simulink model "LV25P_start"  (R2020b)
settings: Solver=VariableStepAuto  StartTime=0.0  StopTime=1/15  RelTol=1e-3
libraries: fl_lib x42, nesl_utility x17
settings Model: Creator=MrNobody  LastModifiedBy=david

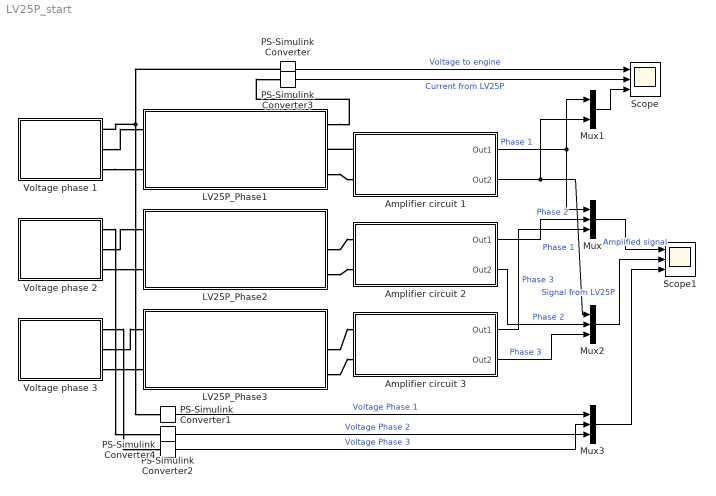
== system LV25P_start ==
  Amplifier circuit 1 : Subsystem
  Amplifier circuit 2 : Subsystem
  Amplifier circuit 3 : Subsystem
  LV25P_Phase1 : Subsystem
  LV25P_Phase2 : Subsystem
  LV25P_Phase3 : Subsystem
  Mux : Mux  Inputs=3
  Mux1 : Mux  Inputs=2
  Mux2 : Mux  Inputs=3
  Mux3 : Mux  Inputs=3
  PS-Simulink Converter{,1..4} (5 alike) : nesl_utility/PS-Simulink Converter  PhysicalDomain=network_engine_domain  SubClassName=ps_output  LeftPortType=input  RightPortType=output  PseudoPeriodic=off  Frequencies=[]  Unit=inherit  AffineConversion=off
  Scope : Scope  NumInputPorts=3
  Scope1 : Scope  NumInputPorts=3
  Voltage phase 1 : Subsystem
  Voltage phase 2 : Subsystem
  Voltage phase 3 : Subsystem
  wires:
  PS-Simulink Converter/1 -> Scope/1  "Voltage to engine"
  PS-Simulink Converter3/1 -> Scope/2  "Current from LV25P"
  Amplifier circuit 1/1(Out1) -> Mux1/1, Mux/1  "Phase 1"
  Amplifier circuit 2/1(Out1) -> Mux/2  "Phase 2"
  Amplifier circuit 3/1(Out1) -> Mux/3  "Phase 3"
  Mux/1 -> Scope1/1  "Amplified signal"
  Amplifier circuit 1/2(Out2) -> Mux2/1, Mux1/2  "Phase 1"
  Mux1/1 -> Scope/3
  Amplifier circuit 2/2(Out2) -> Mux2/2  "Phase 2"
  Amplifier circuit 3/2(Out2) -> Mux2/3  "Phase 3"
  Mux2/1 -> Scope1/2  "Signal from LV25P"
  PS-Simulink Converter4/1 -> Mux3/3  "Voltage Phase 3"
  PS-Simulink Converter2/1 -> Mux3/2  "Voltage Phase 2"
  PS-Simulink Converter1/1 -> Mux3/1  "Voltage Phase 1"
  Mux3/1 -> Scope1/3
  connections:
  PS-Simulink Converter/LConn1 -- Voltage phase 1/RConn1 -- PS-Simulink Converter1/LConn1
  Voltage phase 1/RConn2 -- LV25P_Phase1/LConn1
  Voltage phase 1/RConn3 -- LV25P_Phase1/LConn2
  LV25P_Phase1/RConn1 -- PS-Simulink Converter3/LConn1
  Amplifier circuit 1/LConn1 -- LV25P_Phase1/RConn2
  LV25P_Phase1/RConn3 -- Amplifier circuit 1/LConn2
  Voltage phase 2/RConn2 -- LV25P_Phase2/LConn1
  Voltage phase 2/RConn3 -- LV25P_Phase2/LConn2
  Voltage phase 3/RConn2 -- LV25P_Phase3/LConn1
  Voltage phase 3/RConn3 -- LV25P_Phase3/LConn2
  LV25P_Phase2/RConn2 -- Amplifier circuit 2/LConn1
  LV25P_Phase2/RConn3 -- Amplifier circuit 2/LConn2
  LV25P_Phase3/RConn2 -- Amplifier circuit 3/LConn1
  LV25P_Phase3/RConn3 -- Amplifier circuit 3/LConn2
  Voltage phase 3/RConn1 -- PS-Simulink Converter4/LConn1
  Voltage phase 2/RConn1 -- PS-Simulink Converter2/LConn1

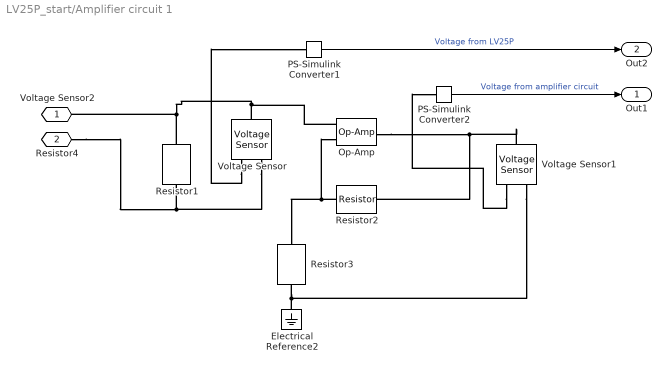
== system LV25P_start/Amplifier circuit 1 ==
  Electrical Reference2 : fl_lib/Electrical/Electrical Elements/Electrical Reference
  Op-Amp : fl_lib/Electrical/Electrical Elements/Op-Amp  outI_specify=off  outI_priority=None  outI=0 A  outI_nominal_specify=off  outI_nominal_unit=A  outI_nominal_value=1
  PS-Simulink Converter1 : nesl_utility/PS-Simulink Converter  PhysicalDomain=network_engine_domain  SubClassName=ps_output  LeftPortType=input  RightPortType=output  PseudoPeriodic=off  Frequencies=[]  Unit=inherit  AffineConversion=off
  PS-Simulink Converter2 : nesl_utility/PS-Simulink Converter  PhysicalDomain=network_engine_domain  SubClassName=ps_output  LeftPortType=input  RightPortType=output  PseudoPeriodic=off  Frequencies=[]  Unit=inherit  AffineConversion=off
  Resistor1 : fl_lib/Electrical/Electrical Elements/Resistor  R=100 Ohm  i_specify=off  i_priority=None  i=0 A  i_nominal_specify=off  i_nominal_unit=A  i_nominal_value=1  v_specify=off  v_priority=None  v=0 V  v_nominal_specify=off  v_nominal_unit=V  v_nominal_value=1
  Resistor2 : fl_lib/Electrical/Electrical Elements/Resistor  R=30 kOhm  i_specify=off  i_priority=None  i=0 A  i_nominal_specify=off  i_nominal_unit=A  i_nominal_value=1  v_specify=off  v_priority=None  v=0 V  v_nominal_specify=off  v_nominal_unit=V  v_nominal_value=1
  Resistor3 : fl_lib/Electrical/Electrical Elements/Resistor  R=10 kOhm  i_specify=off  i_priority=None  i=0 A  i_nominal_specify=off  i_nominal_unit=A  i_nominal_value=1  v_specify=off  v_priority=None  v=0 V  v_nominal_specify=off  v_nominal_unit=V  v_nominal_value=1
  Voltage Sensor : fl_lib/Electrical/Electrical Sensors/Voltage Sensor
  Voltage Sensor1 : fl_lib/Electrical/Electrical Sensors/Voltage Sensor
  Voltage Sensor2 : PMIOPort  Side=Left
  Resistor4 : PMIOPort  Port=2  Side=Left
  Out1 : Outport
  Out2 : Outport  Port=2
  wires:
  PS-Simulink Converter2/1 -> Out1/1  "Voltage from amplifier circuit"
  PS-Simulink Converter1/1 -> Out2/1  "Voltage from LV25P"
  connections:
  Resistor1/LConn1 -- Op-Amp/LConn1 -- Voltage Sensor/LConn1 -- Voltage Sensor2/RConn1
  Op-Amp/RConn1 -- Voltage Sensor1/LConn1 -- Resistor2/RConn1
  Voltage Sensor/RConn2 -- Resistor4/RConn1 -- Resistor1/RConn1
  Voltage Sensor1/RConn1 -- PS-Simulink Converter2/LConn1
  Electrical Reference2/LConn1 -- Voltage Sensor1/RConn2 -- Resistor3/RConn1
  Resistor2/LConn1 -- Op-Amp/LConn2 -- Resistor3/LConn1
  Voltage Sensor/RConn1 -- PS-Simulink Converter1/LConn1

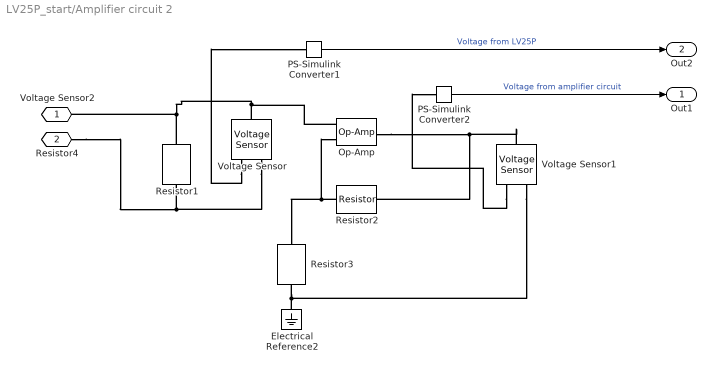
== system LV25P_start/Amplifier circuit 2 ==
  Electrical Reference2 : fl_lib/Electrical/Electrical Elements/Electrical Reference
  Op-Amp : fl_lib/Electrical/Electrical Elements/Op-Amp  outI_specify=off  outI_priority=None  outI=0 A  outI_nominal_specify=off  outI_nominal_unit=A  outI_nominal_value=1
  PS-Simulink Converter1 : nesl_utility/PS-Simulink Converter  PhysicalDomain=network_engine_domain  SubClassName=ps_output  LeftPortType=input  RightPortType=output  PseudoPeriodic=off  Frequencies=[]  Unit=inherit  AffineConversion=off
  PS-Simulink Converter2 : nesl_utility/PS-Simulink Converter  PhysicalDomain=network_engine_domain  SubClassName=ps_output  LeftPortType=input  RightPortType=output  PseudoPeriodic=off  Frequencies=[]  Unit=inherit  AffineConversion=off
  Resistor1 : fl_lib/Electrical/Electrical Elements/Resistor  R=100 Ohm  i_specify=off  i_priority=None  i=0 A  i_nominal_specify=off  i_nominal_unit=A  i_nominal_value=1  v_specify=off  v_priority=None  v=0 V  v_nominal_specify=off  v_nominal_unit=V  v_nominal_value=1
  Resistor2 : fl_lib/Electrical/Electrical Elements/Resistor  R=30 kOhm  i_specify=off  i_priority=None  i=0 A  i_nominal_specify=off  i_nominal_unit=A  i_nominal_value=1  v_specify=off  v_priority=None  v=0 V  v_nominal_specify=off  v_nominal_unit=V  v_nominal_value=1
  Resistor3 : fl_lib/Electrical/Electrical Elements/Resistor  R=10 kOhm  i_specify=off  i_priority=None  i=0 A  i_nominal_specify=off  i_nominal_unit=A  i_nominal_value=1  v_specify=off  v_priority=None  v=0 V  v_nominal_specify=off  v_nominal_unit=V  v_nominal_value=1
  Voltage Sensor : fl_lib/Electrical/Electrical Sensors/Voltage Sensor
  Voltage Sensor1 : fl_lib/Electrical/Electrical Sensors/Voltage Sensor
  Voltage Sensor2 : PMIOPort  Side=Left
  Resistor4 : PMIOPort  Port=2  Side=Left
  Out1 : Outport
  Out2 : Outport  Port=2
  wires:
  PS-Simulink Converter2/1 -> Out1/1  "Voltage from amplifier circuit"
  PS-Simulink Converter1/1 -> Out2/1  "Voltage from LV25P"
  connections:
  Op-Amp/LConn1 -- Voltage Sensor/LConn1 -- Resistor1/LConn1 -- Voltage Sensor2/RConn1
  Op-Amp/RConn1 -- Voltage Sensor1/LConn1 -- Resistor2/RConn1
  Voltage Sensor/RConn2 -- Resistor1/RConn1 -- Resistor4/RConn1
  Voltage Sensor1/RConn1 -- PS-Simulink Converter2/LConn1
  Electrical Reference2/LConn1 -- Voltage Sensor1/RConn2 -- Resistor3/RConn1
  Resistor2/LConn1 -- Op-Amp/LConn2 -- Resistor3/LConn1
  Voltage Sensor/RConn1 -- PS-Simulink Converter1/LConn1

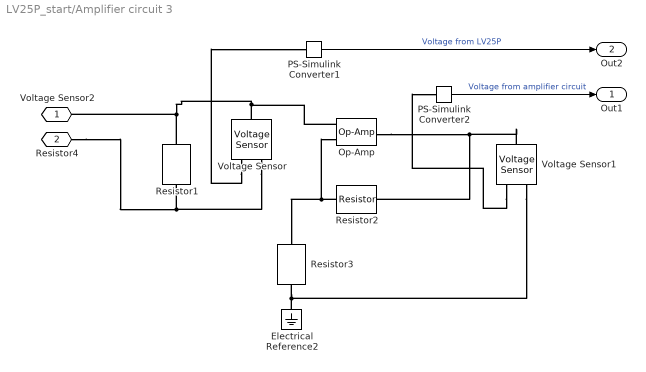
== system LV25P_start/Amplifier circuit 3 ==
  Electrical Reference2 : fl_lib/Electrical/Electrical Elements/Electrical Reference
  Op-Amp : fl_lib/Electrical/Electrical Elements/Op-Amp  outI_specify=off  outI_priority=None  outI=0 A  outI_nominal_specify=off  outI_nominal_unit=A  outI_nominal_value=1
  PS-Simulink Converter1 : nesl_utility/PS-Simulink Converter  PhysicalDomain=network_engine_domain  SubClassName=ps_output  LeftPortType=input  RightPortType=output  PseudoPeriodic=off  Frequencies=[]  Unit=inherit  AffineConversion=off
  PS-Simulink Converter2 : nesl_utility/PS-Simulink Converter  PhysicalDomain=network_engine_domain  SubClassName=ps_output  LeftPortType=input  RightPortType=output  PseudoPeriodic=off  Frequencies=[]  Unit=inherit  AffineConversion=off
  Resistor1 : fl_lib/Electrical/Electrical Elements/Resistor  R=100 Ohm  i_specify=off  i_priority=None  i=0 A  i_nominal_specify=off  i_nominal_unit=A  i_nominal_value=1  v_specify=off  v_priority=None  v=0 V  v_nominal_specify=off  v_nominal_unit=V  v_nominal_value=1
  Resistor2 : fl_lib/Electrical/Electrical Elements/Resistor  R=30 kOhm  i_specify=off  i_priority=None  i=0 A  i_nominal_specify=off  i_nominal_unit=A  i_nominal_value=1  v_specify=off  v_priority=None  v=0 V  v_nominal_specify=off  v_nominal_unit=V  v_nominal_value=1
  Resistor3 : fl_lib/Electrical/Electrical Elements/Resistor  R=10 kOhm  i_specify=off  i_priority=None  i=0 A  i_nominal_specify=off  i_nominal_unit=A  i_nominal_value=1  v_specify=off  v_priority=None  v=0 V  v_nominal_specify=off  v_nominal_unit=V  v_nominal_value=1
  Voltage Sensor : fl_lib/Electrical/Electrical Sensors/Voltage Sensor
  Voltage Sensor1 : fl_lib/Electrical/Electrical Sensors/Voltage Sensor
  Voltage Sensor2 : PMIOPort  Side=Left
  Resistor4 : PMIOPort  Port=2  Side=Left
  Out1 : Outport
  Out2 : Outport  Port=2
  wires:
  PS-Simulink Converter2/1 -> Out1/1  "Voltage from amplifier circuit"
  PS-Simulink Converter1/1 -> Out2/1  "Voltage from LV25P"
  connections:
  Op-Amp/LConn1 -- Voltage Sensor/LConn1 -- Resistor1/LConn1 -- Voltage Sensor2/RConn1
  Op-Amp/RConn1 -- Voltage Sensor1/LConn1 -- Resistor2/RConn1
  Voltage Sensor/RConn2 -- Resistor1/RConn1 -- Resistor4/RConn1
  Voltage Sensor1/RConn1 -- PS-Simulink Converter2/LConn1
  Electrical Reference2/LConn1 -- Voltage Sensor1/RConn2 -- Resistor3/RConn1
  Resistor2/LConn1 -- Op-Amp/LConn2 -- Resistor3/LConn1
  Voltage Sensor/RConn1 -- PS-Simulink Converter1/LConn1

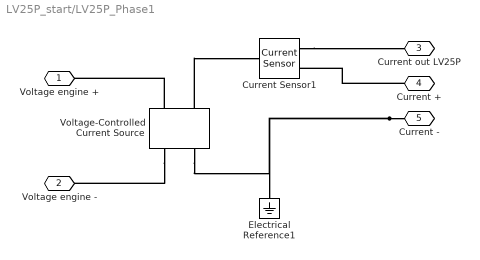
== system LV25P_start/LV25P_Phase1 ==
  Current Sensor1 : fl_lib/Electrical/Electrical Sensors/Current Sensor
  Electrical Reference1 : fl_lib/Electrical/Electrical Elements/Electrical Reference
  Voltage-Controlled Current Source : fl_lib/Electrical/Electrical Sources/Voltage-Controlled Current Source  K=0.000125 1/Ohm  v1_specify=off  v1_priority=None  v1=0 V  v1_nominal_specify=off  v1_nominal_unit=V  v1_nominal_value=1  i2_specify=off  i2_priority=None  i2=0 A  i2_nominal_specify=off  i2_nominal_unit=A  i2_nominal_value=1
      settings: SourceProductBaseCode=SS  InternalSimscapePortConfiguration="{\"Bottom\":[],\"Left\":[{\"id\":\"p1\",\"label\":\"+\",\"type\":\"foundation.electrical.electrical\"},{\"id\":\"head\",\"label\":\"\",\"type\":\"foundation.electrical.electrical\"}],\"Right\":[{\"id\":\"n1\",\"label\":\"-\",\"type\":\"foundation.electrical.electrical\"},{\"id\":\"tail\",\"label\":\"\",\"type\":\"foundation.electrical.electrical\"}],\"Top\":[]}"
  Voltage engine + : PMIOPort  Side=Left
  Voltage engine - : PMIOPort  Port=2  Side=Left
  Current out LV25P : PMIOPort  Port=3  Side=Right
  Current + : PMIOPort  Port=4  Side=Right
  Current - : PMIOPort  Port=5  Side=Right
  connections:
  Current -/RConn1 -- Voltage-Controlled Current Source/RConn2 -- Electrical Reference1/LConn1
  Voltage-Controlled Current Source/LConn2 -- Current Sensor1/LConn1
  Current +/RConn1 -- Current Sensor1/RConn2
  Voltage-Controlled Current Source/RConn1 -- Voltage engine -/RConn1
  Current Sensor1/RConn1 -- Current out LV25P/RConn1
  Voltage-Controlled Current Source/LConn1 -- Voltage engine +/RConn1

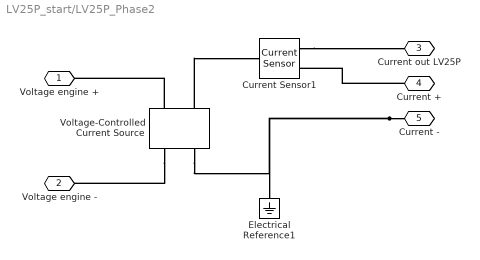
== system LV25P_start/LV25P_Phase2 ==
  Current Sensor1 : fl_lib/Electrical/Electrical Sensors/Current Sensor
  Electrical Reference1 : fl_lib/Electrical/Electrical Elements/Electrical Reference
  Voltage-Controlled Current Source : fl_lib/Electrical/Electrical Sources/Voltage-Controlled Current Source  K=0.000125 1/Ohm  v1_specify=off  v1_priority=None  v1=0 V  v1_nominal_specify=off  v1_nominal_unit=V  v1_nominal_value=1  i2_specify=off  i2_priority=None  i2=0 A  i2_nominal_specify=off  i2_nominal_unit=A  i2_nominal_value=1
      settings: SourceProductBaseCode=SS  InternalSimscapePortConfiguration="{\"Bottom\":[],\"Left\":[{\"id\":\"p1\",\"label\":\"+\",\"type\":\"foundation.electrical.electrical\"},{\"id\":\"head\",\"label\":\"\",\"type\":\"foundation.electrical.electrical\"}],\"Right\":[{\"id\":\"n1\",\"label\":\"-\",\"type\":\"foundation.electrical.electrical\"},{\"id\":\"tail\",\"label\":\"\",\"type\":\"foundation.electrical.electrical\"}],\"Top\":[]}"
  Voltage engine + : PMIOPort  Side=Left
  Voltage engine - : PMIOPort  Port=2  Side=Left
  Current out LV25P : PMIOPort  Port=3  Side=Right
  Current + : PMIOPort  Port=4  Side=Right
  Current - : PMIOPort  Port=5  Side=Right
  connections:
  Current -/RConn1 -- Electrical Reference1/LConn1 -- Voltage-Controlled Current Source/RConn2
  Voltage-Controlled Current Source/LConn2 -- Current Sensor1/LConn1
  Current +/RConn1 -- Current Sensor1/RConn2
  Voltage-Controlled Current Source/RConn1 -- Voltage engine -/RConn1
  Current Sensor1/RConn1 -- Current out LV25P/RConn1
  Voltage-Controlled Current Source/LConn1 -- Voltage engine +/RConn1

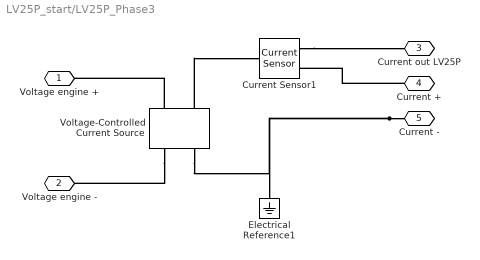
== system LV25P_start/LV25P_Phase3 ==
  Current Sensor1 : fl_lib/Electrical/Electrical Sensors/Current Sensor
  Electrical Reference1 : fl_lib/Electrical/Electrical Elements/Electrical Reference
  Voltage-Controlled Current Source : fl_lib/Electrical/Electrical Sources/Voltage-Controlled Current Source  K=0.000125 1/Ohm  v1_specify=off  v1_priority=None  v1=0 V  v1_nominal_specify=off  v1_nominal_unit=V  v1_nominal_value=1  i2_specify=off  i2_priority=None  i2=0 A  i2_nominal_specify=off  i2_nominal_unit=A  i2_nominal_value=1
      settings: SourceProductBaseCode=SS  InternalSimscapePortConfiguration="{\"Bottom\":[],\"Left\":[{\"id\":\"p1\",\"label\":\"+\",\"type\":\"foundation.electrical.electrical\"},{\"id\":\"head\",\"label\":\"\",\"type\":\"foundation.electrical.electrical\"}],\"Right\":[{\"id\":\"n1\",\"label\":\"-\",\"type\":\"foundation.electrical.electrical\"},{\"id\":\"tail\",\"label\":\"\",\"type\":\"foundation.electrical.electrical\"}],\"Top\":[]}"
  Voltage engine + : PMIOPort  Side=Left
  Voltage engine - : PMIOPort  Port=2  Side=Left
  Current out LV25P : PMIOPort  Port=3  Side=Right
  Current + : PMIOPort  Port=4  Side=Right
  Current - : PMIOPort  Port=5  Side=Right
  connections:
  Current -/RConn1 -- Electrical Reference1/LConn1 -- Voltage-Controlled Current Source/RConn2
  Voltage-Controlled Current Source/LConn2 -- Current Sensor1/LConn1
  Current +/RConn1 -- Current Sensor1/RConn2
  Voltage-Controlled Current Source/RConn1 -- Voltage engine -/RConn1
  Current Sensor1/RConn1 -- Current out LV25P/RConn1
  Voltage-Controlled Current Source/LConn1 -- Voltage engine +/RConn1

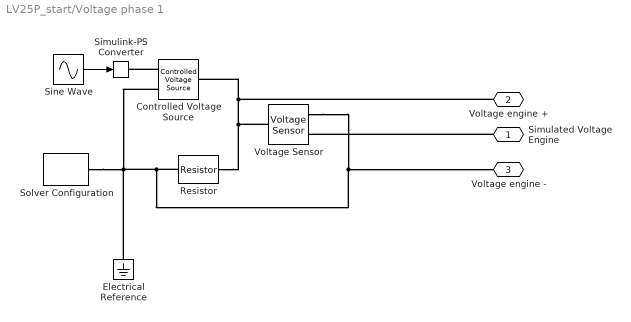
== system LV25P_start/Voltage phase 1 ==
  Controlled Voltage Source : fl_lib/Electrical/Electrical Sources/Controlled Voltage Source
  Electrical Reference : fl_lib/Electrical/Electrical Elements/Electrical Reference
  Resistor : fl_lib/Electrical/Electrical Elements/Resistor  R=10 Ohm  i_specify=off  i_priority=None  i=0 A  i_nominal_specify=off  i_nominal_unit=A  i_nominal_value=1  v_specify=off  v_priority=None  v=0 V  v_nominal_specify=off  v_nominal_unit=V  v_nominal_value=1
  Simulink-PS Converter : nesl_utility/Simulink-PS Converter  PhysicalDomain=network_engine_domain  SubClassName=ps_input  LeftPortType=input  RightPortType=output  PseudoPeriodic=off  Frequencies=[]  NoiseDistribution=none  NoiseParameters=[]  Unit=1  AffineConversion=off  FilteringAndDerivatives=provide  SimscapeFilterOrder=1  InputFilterTimeConstant=0.001  UdotUserProvided=0
  Sine Wave : Sin  Amplitude=200  Frequency=200  SampleTime=0
  Solver Configuration : nesl_utility/Solver Configuration  PhysicalDomain=network_engine_domain  SubClassName=solver  LeftPortType=input  RightPortType=generic  Tones=[]  Harmonics=[]  SimulateNoise=off  Profile=off  UseLocalSampling=off  EnableSwitchedLinearOptims=on  FrequencyDomain=off  UseCCode=off  RelTol=0.001  AbsTol=1e-06  MinStep=1e-09  ToWorkspace=off  RevertToSquareIcSolve=off  NumHomotopyIterations=100  PhasorMode=off  PhasorModeNumHarmonics=1  DoDC=off  ResidualTolerance=1e-09  UseLocalSolver=off  LocalSolverChoice=NE_BACKWARD_EULER_ADVANCER  LocalSolverSampleTime=0.001  DoFixedCost=off  MaxNonlinIter=3  MaxModeIter=2  ComputeImpulses=off  ImpulseIterations=2  LinearAlgebra=auto  EquationFormulation=NE_TIME_EF  DelaysMemoryBudget=1024  AutomaticFiltering=on  FilteringTimeConstant=0.001  PartitionStorageMethod=AS_NEEDED  PartitionMemoryBudget=1024  PartitionMethod=ROBUST
  Voltage Sensor : fl_lib/Electrical/Electrical Sensors/Voltage Sensor
  Simulated Voltage Engine : PMIOPort  Side=Right
  Voltage engine + : PMIOPort  Port=2  Side=Right
  Voltage engine - : PMIOPort  Port=3  Side=Right
  wires:
  Sine Wave/1 -> Simulink-PS Converter/1
  connections:
  Controlled Voltage Source/RConn1 -- Simulink-PS Converter/RConn1
  Simulated Voltage Engine/RConn1 -- Voltage Sensor/RConn1
  Voltage Sensor/LConn1 -- Controlled Voltage Source/LConn1 -- Voltage engine +/RConn1 -- Resistor/RConn1
  Resistor/LConn1 -- Voltage Sensor/RConn2 -- Voltage engine -/RConn1 -- Electrical Reference/LConn1 -- Solver Configuration/RConn1 -- Controlled Voltage Source/RConn2

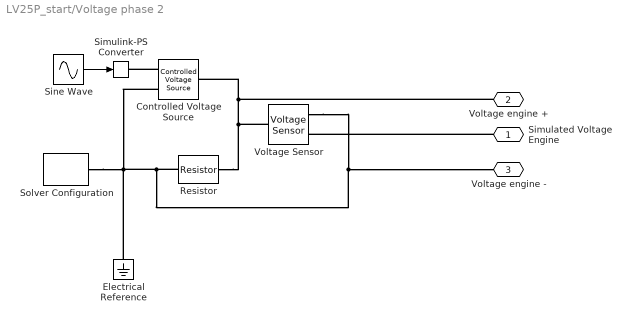
== system LV25P_start/Voltage phase 2 ==
  Controlled Voltage Source : fl_lib/Electrical/Electrical Sources/Controlled Voltage Source
  Electrical Reference : fl_lib/Electrical/Electrical Elements/Electrical Reference
  Resistor : fl_lib/Electrical/Electrical Elements/Resistor  R=10 Ohm  i_specify=off  i_priority=None  i=0 A  i_nominal_specify=off  i_nominal_unit=A  i_nominal_value=1  v_specify=off  v_priority=None  v=0 V  v_nominal_specify=off  v_nominal_unit=V  v_nominal_value=1
  Simulink-PS Converter : nesl_utility/Simulink-PS Converter  PhysicalDomain=network_engine_domain  SubClassName=ps_input  LeftPortType=input  RightPortType=output  PseudoPeriodic=off  Frequencies=[]  NoiseDistribution=none  NoiseParameters=[]  Unit=1  AffineConversion=off  FilteringAndDerivatives=provide  SimscapeFilterOrder=1  InputFilterTimeConstant=0.001  UdotUserProvided=0
  Sine Wave : Sin  Amplitude=200  Frequency=200  Phase=2*pi/3  SampleTime=0
  Solver Configuration : nesl_utility/Solver Configuration  PhysicalDomain=network_engine_domain  SubClassName=solver  LeftPortType=input  RightPortType=generic  Tones=[]  Harmonics=[]  SimulateNoise=off  Profile=off  UseLocalSampling=off  EnableSwitchedLinearOptims=on  FrequencyDomain=off  UseCCode=off  RelTol=0.001  AbsTol=1e-06  MinStep=1e-09  ToWorkspace=off  RevertToSquareIcSolve=off  NumHomotopyIterations=100  PhasorMode=off  PhasorModeNumHarmonics=1  DoDC=off  ResidualTolerance=1e-09  UseLocalSolver=off  LocalSolverChoice=NE_BACKWARD_EULER_ADVANCER  LocalSolverSampleTime=0.001  DoFixedCost=off  MaxNonlinIter=3  MaxModeIter=2  ComputeImpulses=off  ImpulseIterations=2  LinearAlgebra=auto  EquationFormulation=NE_TIME_EF  DelaysMemoryBudget=1024  AutomaticFiltering=on  FilteringTimeConstant=0.001  PartitionStorageMethod=AS_NEEDED  PartitionMemoryBudget=1024  PartitionMethod=ROBUST
  Voltage Sensor : fl_lib/Electrical/Electrical Sensors/Voltage Sensor
  Simulated Voltage Engine : PMIOPort  Side=Right
  Voltage engine + : PMIOPort  Port=2  Side=Right
  Voltage engine - : PMIOPort  Port=3  Side=Right
  wires:
  Sine Wave/1 -> Simulink-PS Converter/1
  connections:
  Controlled Voltage Source/RConn1 -- Simulink-PS Converter/RConn1
  Simulated Voltage Engine/RConn1 -- Voltage Sensor/RConn1
  Resistor/RConn1 -- Voltage Sensor/LConn1 -- Voltage engine +/RConn1 -- Controlled Voltage Source/LConn1
  Electrical Reference/LConn1 -- Solver Configuration/RConn1 -- Controlled Voltage Source/RConn2 -- Resistor/LConn1 -- Voltage engine -/RConn1 -- Voltage Sensor/RConn2

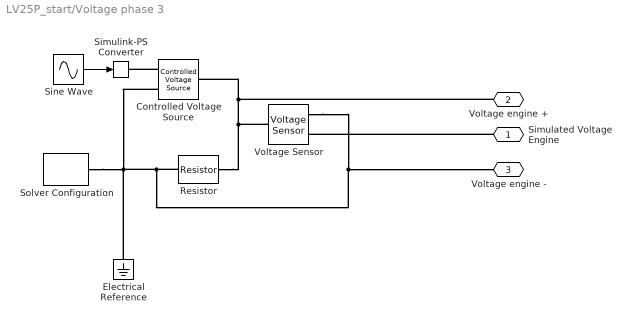
== system LV25P_start/Voltage phase 3 ==
  Controlled Voltage Source : fl_lib/Electrical/Electrical Sources/Controlled Voltage Source
  Electrical Reference : fl_lib/Electrical/Electrical Elements/Electrical Reference
  Resistor : fl_lib/Electrical/Electrical Elements/Resistor  R=10 Ohm  i_specify=off  i_priority=None  i=0 A  i_nominal_specify=off  i_nominal_unit=A  i_nominal_value=1  v_specify=off  v_priority=None  v=0 V  v_nominal_specify=off  v_nominal_unit=V  v_nominal_value=1
  Simulink-PS Converter : nesl_utility/Simulink-PS Converter  PhysicalDomain=network_engine_domain  SubClassName=ps_input  LeftPortType=input  RightPortType=output  PseudoPeriodic=off  Frequencies=[]  NoiseDistribution=none  NoiseParameters=[]  Unit=1  AffineConversion=off  FilteringAndDerivatives=provide  SimscapeFilterOrder=1  InputFilterTimeConstant=0.001  UdotUserProvided=0
  Sine Wave : Sin  Amplitude=200  Frequency=200  Phase=4*pi/3  SampleTime=0
  Solver Configuration : nesl_utility/Solver Configuration  PhysicalDomain=network_engine_domain  SubClassName=solver  LeftPortType=input  RightPortType=generic  Tones=[]  Harmonics=[]  SimulateNoise=off  Profile=off  UseLocalSampling=off  EnableSwitchedLinearOptims=on  FrequencyDomain=off  UseCCode=off  RelTol=0.001  AbsTol=1e-06  MinStep=1e-09  ToWorkspace=off  RevertToSquareIcSolve=off  NumHomotopyIterations=100  PhasorMode=off  PhasorModeNumHarmonics=1  DoDC=off  ResidualTolerance=1e-09  UseLocalSolver=off  LocalSolverChoice=NE_BACKWARD_EULER_ADVANCER  LocalSolverSampleTime=0.001  DoFixedCost=off  MaxNonlinIter=3  MaxModeIter=2  ComputeImpulses=off  ImpulseIterations=2  LinearAlgebra=auto  EquationFormulation=NE_TIME_EF  DelaysMemoryBudget=1024  AutomaticFiltering=on  FilteringTimeConstant=0.001  PartitionStorageMethod=AS_NEEDED  PartitionMemoryBudget=1024  PartitionMethod=ROBUST
  Voltage Sensor : fl_lib/Electrical/Electrical Sensors/Voltage Sensor
  Simulated Voltage Engine : PMIOPort  Side=Right
  Voltage engine + : PMIOPort  Port=2  Side=Right
  Voltage engine - : PMIOPort  Port=3  Side=Right
  wires:
  Sine Wave/1 -> Simulink-PS Converter/1
  connections:
  Controlled Voltage Source/RConn1 -- Simulink-PS Converter/RConn1
  Simulated Voltage Engine/RConn1 -- Voltage Sensor/RConn1
  Resistor/RConn1 -- Voltage Sensor/LConn1 -- Voltage engine +/RConn1 -- Controlled Voltage Source/LConn1
  Electrical Reference/LConn1 -- Solver Configuration/RConn1 -- Controlled Voltage Source/RConn2 -- Resistor/LConn1 -- Voltage engine -/RConn1 -- Voltage Sensor/RConn2
